simulink model "ECE125FinalProjectStatespace"  (R2025a)
settings: Solver=FixedStepAuto  StartTime=0.0  StopTime=40  FixedStep=5e-3  RelTol=1e-3
settings Model: Creator=frank  LastModifiedBy=frank

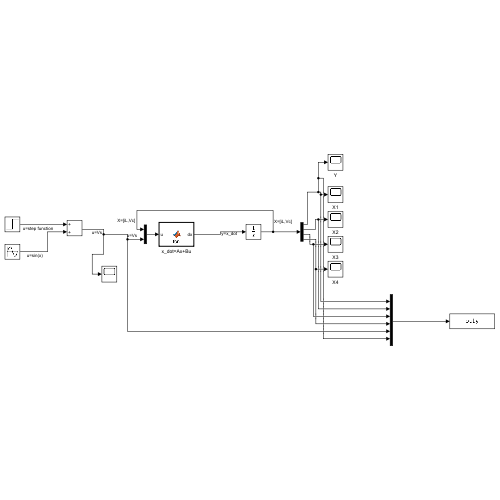
[thumbnail: Simulink's stored preview of the top-level diagram]
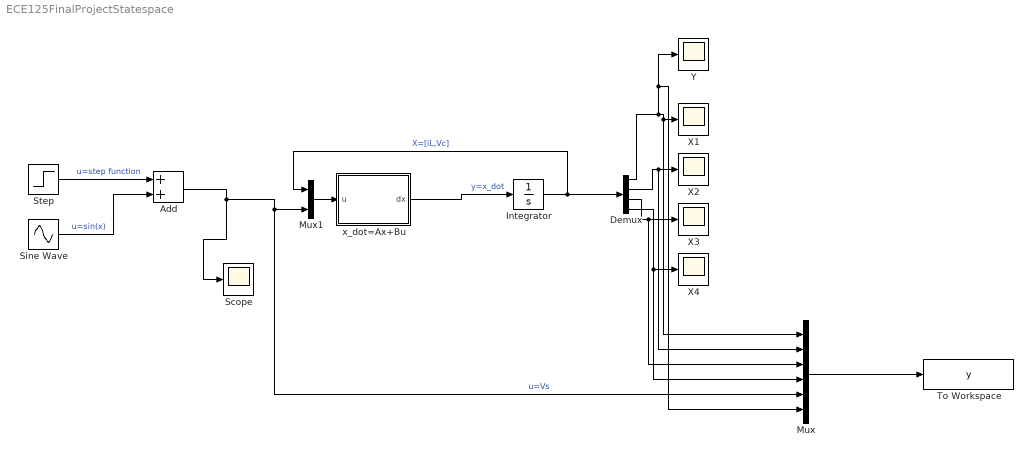
== system ECE125FinalProjectStatespace ==
  Add : Sum
  Demux : Demux
  Integrator : Integrator  InitialCondition=[0;0;0;0]+1
  Mux : Mux  Inputs=6
  Mux1 : Mux  Inputs=2
  Scope : Scope
      settings: ActiveDisplayYMinimum=-1  ActiveDisplayYMaximum=1  DataLoggingVariableName=ScopeData5
  Sine Wave : Sin  Frequency=3  SampleTime=0
  Step : Step  After=100  SampleTime=0
  To Workspace : ToWorkspace  VariableName=y  SampleTime=-1
  X{1..4} (4 alike) : Scope
      X1 settings: ActiveDisplayYMinimum=-1  ActiveDisplayYMaximum=1
      X2 settings: ActiveDisplayYMinimum=-0.731082516340076  ActiveDisplayYMaximum=2.5700109526448909
      X3 settings: ActiveDisplayYMinimum=-4.2338617490379846  ActiveDisplayYMaximum=5.2769646619809807  DataLoggingVariableName=ScopeData2
      X4 settings: ActiveDisplayYMinimum=-40.10391894281878  ActiveDisplayYMaximum=56.401301426050537  DataLoggingVariableName=ScopeData3
  Y : Scope
      settings: ActiveDisplayYMinimum=-1  ActiveDisplayYMaximum=1  DataLoggingVariableName=ScopeData4
  x_dot=Ax+Bu : MATLAB Function  TreatAsAtomicUnit=on
  wires:
  Add/1 -> Scope/1, Mux/5, Mux1/2  "u=Vs"
  x_dot=Ax+Bu/1(dx) -> Integrator/1  "y=x_dot"
  Integrator/1 -> Mux1/1, Demux/1  "X=[iL,Vc]"
  Demux/1 -> Y/1, Mux/6, Mux/1, X1/1
  Demux/2 -> Mux/2, X2/1
  Demux/3 -> X3/1, Mux/3
  Demux/4 -> Mux/4, X4/1
  Mux/1 -> To Workspace/1
  Mux1/1 -> x_dot=Ax+Bu/1(u)
  Step/1 -> Add/1  "u=step function"
  Sine Wave/1 -> Add/2  "u=sin(x)"

== matlab function ECE125FinalProjectStatespace/x_dot=Ax+Bu ==
  data: u input; dx output
function dx = fcn(u) 
x = u(1:4);
u_in = u(5);
A=[0 1 0 0;
   0 0 1 0;
   0 0 0 1;
  -24 -50 -35 -10];
B=[0;0;0;1];
dx=A*x+B*u_in;
end
